simulink model "ekfPacked"  (R2019b)
settings: Solver=VariableStepAuto  StartTime=0.0  StopTime=10.0  RelTol=1e-3
settings Model: Creator=Alireza  LastModifiedBy=Alireza

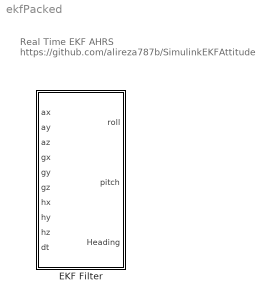
== system ekfPacked ==
  note: Real Time EKF AHRS
      | https://github.com/alireza787b/SimulinkEKFAttitude
  EKF Filter : Subsystem

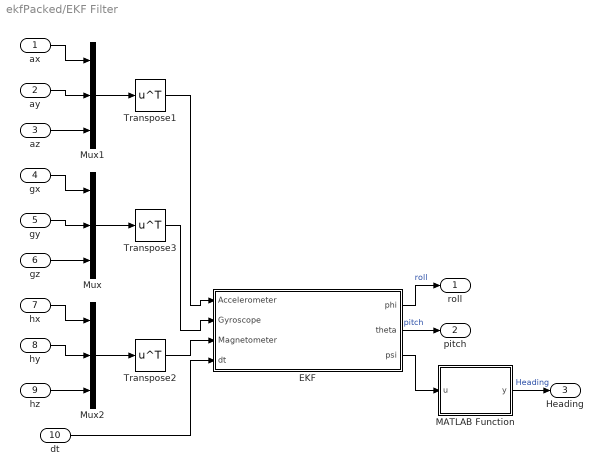
== system ekfPacked/EKF Filter ==
  ax : Inport
  ay : Inport  Port=2
  az : Inport  Port=3
  gx : Inport  Port=4
  gy : Inport  Port=5
  gz : Inport  Port=6
  hx : Inport  Port=7
  hy : Inport  Port=8
  hz : Inport  Port=9
  dt : Inport  Port=10
  EKF : MATLAB Function  TreatAsAtomicUnit=on
  MATLAB Function : MATLAB Function  TreatAsAtomicUnit=on
  Mux : Mux  Inputs=3
  Mux1 : Mux  Inputs=3
  Mux2 : Mux  Inputs=3
  Transpose1 : Math  Operator=transpose  SaturateOnIntegerOverflow=on
  Transpose2 : Math  Operator=transpose  SaturateOnIntegerOverflow=on
  Transpose3 : Math  Operator=transpose  SaturateOnIntegerOverflow=on
  roll : Outport
  pitch : Outport  Port=2
  Heading : Outport  Port=3
  wires:
  MATLAB Function/1(y) -> Heading/1  "Heading"
  gy/1 -> Mux/2
  gz/1 -> Mux/3
  hz/1 -> Mux2/3
  ax/1 -> Mux1/1
  az/1 -> Mux1/3
  EKF/1(phi) -> roll/1  "roll"
  ay/1 -> Mux1/2
  Mux2/1 -> Transpose2/1
  Transpose1/1 -> EKF/1(Accelerometer)
  hx/1 -> Mux2/1
  Transpose2/1 -> EKF/3(Magnetometer)
  Mux1/1 -> Transpose1/1
  Mux/1 -> Transpose3/1
  EKF/3(psi) -> MATLAB Function/1(u)
  EKF/2(theta) -> pitch/1  "pitch"
  gx/1 -> Mux/1
  hy/1 -> Mux2/2
  Transpose3/1 -> EKF/2(Gyroscope)
  dt/1 -> EKF/4(dt)

== matlab function ekfPacked/EKF Filter/EKF ==
  data: Accelerometer input; phi output; Gyroscope input; Magnetometer input; theta output; psi output; dt input
function [phi, theta, psi] = fcn(Accelerometer,Gyroscope,Magnetometer,dt)
persistent AHRSEKF;
if isempty(AHRSEKF)
    AHRSEKF = EKFfilter();
end
    AHRSEKF.Update(dt, Gyroscope(1,:) , Accelerometer(1,:), Magnetometer(1,:));
     phi = AHRSEKF.eulerAngles(1,1);   
     theta = AHRSEKF.eulerAngles(2,1);   
     psi = AHRSEKF.eulerAngles(3,1); 

end

== matlab function ekfPacked/EKF Filter/MATLAB Function ==
  data: u input; y output
function y = angleCorrection(u)
if u<0
    y = u+6.2832;

else
y = u;
end 
end
